simulink model "Accelerometer_model"  (R2015a)
settings: Solver=ode45  StartTime=0.0  StopTime=10.0  RelTol=1e-3
InitFcn:
  | Accelerometer_config;
undefined symbols (not defined in the file or in its folder): accelerometer
settings Model: Creator=hamada  LastModifiedBy=hamada

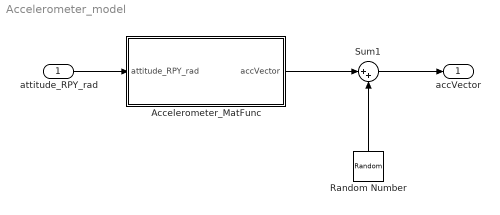
== system Accelerometer_model ==
  attitude_RPY_rad : Inport  PortDimensions=3
  Accelerometer_MatFunc : MATLAB Function  TreatAsAtomicUnit=on
  Random Number : RandomNumber  Mean=accelerometer.bias  Variance=accelerometer.variant  SampleTime=accelerometer.period
  Sum1 : Sum  Inputs=|++
  accVector : Outport
  wires:
  attitude_RPY_rad/1 -> Accelerometer_MatFunc/1(attitude_RPY_rad)
  Accelerometer_MatFunc/1(accVector) -> Sum1/1
  Sum1/1 -> accVector/1
  Random Number/1 -> Sum1/2

== matlab function Accelerometer_model/Accelerometer_MatFunc ==
  data: attitude_RPY_rad input; accVector output
function accVector = Accelerometer_MatFunc( attitude_RPY_rad )
    %#codegen
    accVector = Accelerometer( attitude_RPY_rad  );
end
